simulink library "calcFluidDynamicLoads_hydroelasticVersion"  (R2022a)
settings: Solver=VariableStepAuto  StartTime=0.0  StopTime=10.0  RelTol=1e-3
values from neighbouring files (symbols this model uses):
  fluidDensity = 1000    [fluidDynamicSurface_ts.m]
undefined symbols (not defined in the file or in its folder): base_checkBending, base_checkTwisting, Copy_of_clAndCdCalculator_cl, E_matlabEnv, fluidMomentArms, fluidRefArea, G_matlabEnv, rho, Subsystem, vcl, vhcl, wingTips
libraries: dspstat3 x4, dsppolyfun x4, vrlib x3, dynamicPressure_ul x1, eeGeneralControl x1, alphaBetaLE_ul x1, localApparentWind_ul x1, rotateAboutVec x1, wingAnalysis_stateflow x1
settings Model: Creator=Ayaz  LastModifiedBy=Carson
settings SolverCC: AlgebraicLoopSolver=TrustRegion
settings DebuggingCC: UnconnectedInputMsg=warning  UnconnectedOutputMsg=warning  UnconnectedLineMsg=warning  SFMachineParentedDataDiag=warning

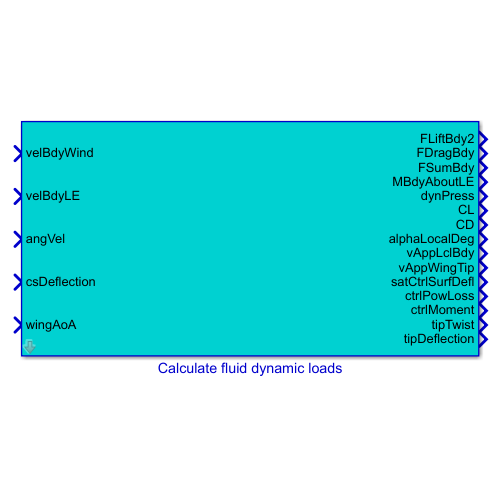
[thumbnail: Simulink's stored preview of the top-level diagram]
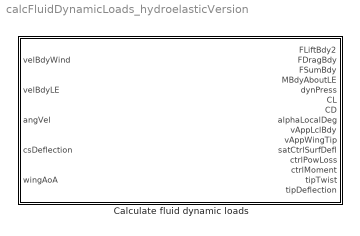
== system calcFluidDynamicLoads_hydroelasticVersion ==
  Calculate fluid dynamic loads : Subsystem  mask{aSurf=vcl.portWing, sRef=fluidRefArea, rArm_LE=fluidMomentArms(:,1), rTip_LE=wingTips(:,1), fluidDensity=fluidDensity}
      mask prompts: aSurf "Aerosurf object"; sRef "Reference area"; rArm_LE "Moment arm wrt wing LE"; rTip_LE "Surface tip wrt wing LE"; fluidDensity "Fluid density"

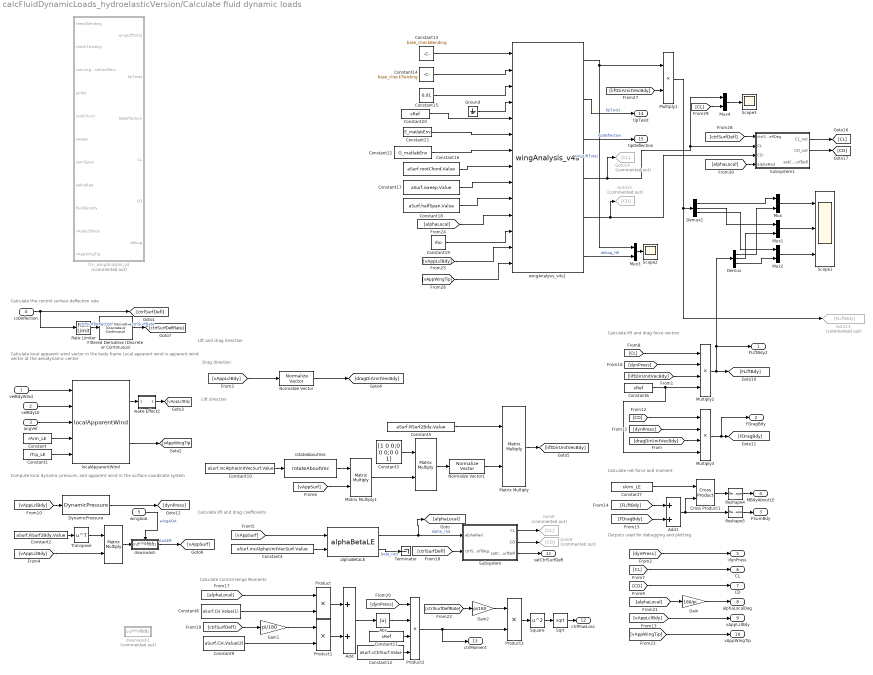
== system calcFluidDynamicLoads_hydroelasticVersion/Calculate fluid dynamic loads ==
  note: Calculate Control Hinge Moments
  note: Calculate the control surface deflection rate
  note: Lift and drag direction
  note: Lift direction
  note: Drag direction
  note: Compute local dynamic pressure,
      | and apparent wind in the surface coordinate system
  note: Calculate local apparent wind vector in the body frame
      | Local apparent wind is apparent wind vector at the aerodynamic center
  note: Calculate lift and drag coefficients
  note: Calculate net force and moment
  note: Outputs used for debugging and plotting.
  note: Calculate lift and drag force vectors
  velBdyWind : Inport
  velBdyLE : Inport  Port=2
  angVel : Inport  Port=3
  csDeflection : Inport  Port=4
  wingAoA : Inport  Port=5
  " " : Product  Multiplication=Matrix(*)
  "  " : Product  Multiplication=Matrix(*)
  Abs : Abs  SaturateOnIntegerOverflow=off
  Add : Sum
  Add1 : Sum
  Constant : Constant  Value=rArm_LE  VectorParams1D=off
  Constant1 : Constant  Value=rTip_LE  VectorParams1D=off
  Constant10 : Constant  Value=aSurf.incAlphaUnitVecSurf.Value  VectorParams1D=off
  Constant11 : Constant  Value=sRef
  Constant12 : Constant  Value=aSurf.cCtrlSurf.Value
  Constant13 : Constant  Value=base_checkBending  OutDataTypeStr=boolean
  Constant14 : Constant  Value=base_checkTwisting  OutDataTypeStr=boolean
  Constant15 : Constant  Value=0.01  OutDataTypeStr=double
  Constant16 : Constant  Value=aSurf.rootChord.Value
  Constant17 : Constant  Value=aSurf.sweep.Value
  Constant18 : Constant  Value=aSurf.halfSpan.Value
  Constant19 : Constant  Value=rho
  Constant2 : Constant  Value=aSurf.RSurf2Bdy.Value  VectorParams1D=off
  Constant20 : Constant  Value=sRef
  Constant21 : Constant  Value=E_matlabEnv
  Constant22 : Constant  Value=G_matlabEnv
  Constant3 : Constant  Value=[1 0 0;0 0 0;0 0 1]  VectorParams1D=off
  Constant4 : Constant  Value=aSurf.incAlphaUnitVecSurf.Value  VectorParams1D=off
  Constant5 : Constant  Value=aSurf.RSurf2Bdy.Value  VectorParams1D=off
  Constant6 : Constant  Value=sRef
  Constant7 : Constant  Value=rArm_LE  VectorParams1D=off
  Constant8 : Constant  Value=aSurf.CH.Value(1)
  Constant9 : Constant  Value=aSurf.CH.Value(2)
  Cross Product1 : vrlib/Utilities/Cross Product
  Demux : Demux  Outputs=3
  Demux1 : Demux  Outputs=3
  DynamicPressure : dynamicPressure_ul/DynamicPressure  rho=fluidDensity
  Filtered Derivative (Discrete or Continuous) : eeGeneralControl/Filtered Derivative (Discrete or Continuous)  K=1  T=.001  B=inf  A=-inf  minRatio=10  init_option=Inherited from block input  x0=0  Ts=-1
      settings: SourceProductBaseCode=PS
  Gain : Gain  Gain=180/pi
  Gain1 : Gain  Gain=pi/180
  Gain2 : Gain  Gain=pi/180
  Goto13 : Goto  Commented=on  GotoTag=FLiftBdy
  Goto14 : Goto  Commented=on  GotoTag=CL
  Goto15 : Goto  Commented=on  GotoTag=CD
  Goto8 : Goto  Commented=on  GotoTag=CL
  Goto9 : Goto  Commented=on  GotoTag=CD
  Ground : Ground
  Matrix Multiply : Product  Multiplication=Matrix(*)
  Matrix Multiply1 : Product  Multiplication=Matrix(*)
  Multiply1 : Product
  Multiply2 : Product  Inputs=4
  Multiply3 : Product  Inputs=4
  Mux{,1..4} (5 alike) : Mux  Inputs=2
  Normalize Vector : vrlib/Utilities/Normalize Vector  maxzero=0
  Normalize Vector1 : vrlib/Utilities/Normalize Vector  maxzero=0
  Product : Product
  Product1 : Product
  Product2 : Product  Inputs=4
  Product3 : Product
  Rate Limiter : RateLimiter  RisingSlewLimit=aSurf.maxCtrlDefSpeed.Value  FallingSlewLimit=-aSurf.maxCtrlDefSpeed.Value  SampleTimeMode=inherited
  Reshape4 : Reshape  OutputDimensionality=Column vector (2-D)
  Reshape5 : Reshape  OutputDimensionality=Column vector (2-D)
  Scope1 : Scope  NumInputPorts=3
  Scope2 : Scope
  Scope3 : Scope
  Sqrt : Sqrt
  Square : Math  Operator=square
  Subsystem : Subsystem  AncestorBlock=Copy_of_clAndCdCalculator_cl/Subsystem  mask{aSurf=aSurf}
      mask prompts: aSurf "aeroSurf object"
  Subsystem1 : Subsystem  mask{aSurf=aSurf}
      mask prompts: aSurf "aeroSurf object"
  Terminator : Terminator
  Transpose : Math  Operator=transpose  SignedPower=on
  alphaBetaLE : alphaBetaLE_ul/alphaBetaLE  SystemSampleTime=-1  VariantActivationTime=update diagram  Latency=0  AutoFrameSizeCalculation=off
  downwash : Subsystem
      settings: PortSchema="{\"entries\":[{\"content\":{\"sides\":[{\"content\":{\"connectorIds\":[\"In1\"]},\"type\":\"ConnectorPlacement.EquallySpacedRectSide\",\"uuid\":\"04ef6d2a-4770-4c63-9c45-9df535824cb6\"},{\"content\":{\"connectorIds\":[\"Out1\"],\"side\":\"RIGHT\"},\"type\":\"ConnectorPlacement.EquallySpacedRectSide\",\"uuid\":\"1e7f53a7-5f70-4bf0-8214-dce734c1b44e\"},{\"content\":{\"connectorIds\":[\"In2\"],\"side\":\"TOP\"},\"type\":\"ConnectorPlacement.EquallySpacedRectSide\",\"uuid\":\"18f507fa-715b-4755-b9b5-759b08e40168\"}]},\"type\":\"ConnectorPlacement.EquallySpacedConnector\",\"uuid\":\"684cff60-c972-427b-b388-36808b9016c1\"}],\"packageUris\":[\"http://schema.mathworks.com/mf0/Connector/19700101\"],\"version\":\"1.0\"}"
  downwash1 : Subsystem  Commented=on
      settings: PortSchema="{\"entries\":[{\"content\":{\"sides\":[{\"content\":{\"connectorIds\":[\"In1\"]},\"type\":\"ConnectorPlacement.EquallySpacedRectSide\",\"uuid\":\"04ef6d2a-4770-4c63-9c45-9df535824cb6\"},{\"content\":{\"connectorIds\":[\"Out1\"],\"side\":\"RIGHT\"},\"type\":\"ConnectorPlacement.EquallySpacedRectSide\",\"uuid\":\"1e7f53a7-5f70-4bf0-8214-dce734c1b44e\"},{\"content\":{\"connectorIds\":[\"In2\"],\"side\":\"TOP\"},\"type\":\"ConnectorPlacement.EquallySpacedRectSide\",\"uuid\":\"18f507fa-715b-4755-b9b5-759b08e40168\"}]},\"type\":\"ConnectorPlacement.EquallySpacedConnector\",\"uuid\":\"684cff60-c972-427b-b388-36808b9016c1\"}],\"packageUris\":[\"http://schema.mathworks.com/mf0/Connector/19700101\"],\"version\":\"1.0\"}"
  fcn_wingAnalysis_v4 : MATLAB Function  Commented=on  TreatAsAtomicUnit=on  SystemSampleTime=0.1
  localApparentWind : localApparentWind_ul/localApparentWind  SystemSampleTime=-1  VariantActivationTime=update diagram  Latency=0  AutoFrameSizeCalculation=off
  rotateAboutVec : rotateAboutVec/rotateAboutVec  ang=90
  wake Effect2 : Subsystem
  wingAnalysis_v4s1 : wingAnalysis_stateflow/wingAnalysis_v4s  SystemSampleTime=-1  VariantActivationTime=update diagram  Latency=0  AutoFrameSizeCalculation=off
      settings: PortSchema="{\"entries\":[{\"content\":{\"sides\":[{\"content\":{\"connectorIds\":[\"In1\",\"In2\",\"In3\",\"In11\",\"In12\",\"In13\",\"In14\",\"In4\",\"In5\",\"In6\",\"In7\",\"In8\",\"In9\",\"In10\"]},\"type\":\"ConnectorPlacement.EquallySpacedRectSide\",\"uuid\":\"6c729b90-d4cd-42cb-9ba5-b5252b1be0f3\"},{\"content\":{\"connectorIds\":[\"Out1\",\"Out2\",\"Out3\",\"Out4\",\"Out5\",\"Out6\"],\"side\":\"RIGHT\"},\"type\":\"ConnectorPlacement.EquallySpacedRectSide\",\"uuid\":\"eea762ff-71d7-4c66-90ee-932d903c73e3\"},{\"content\":{\"connectorIds\":[],\"side\":\"TOP\"},\"type\":\"ConnectorPlacement.EquallySpacedRectSide\",\"uuid\":\"df2db980-21fc-49eb-9688-a3d788e0d700\"}]},\"type\":\"ConnectorPlacement.EquallySpacedConnector\",\"uuid\":\"bf53f703-2290-4676-ac3c-dcfa73901a98\"}],\"packageUris\":[\"http://schema.mathworks.com/mf0/Connector/R2020b\"],\"version\":\"1.0\"}"
  FLiftBdy2 : Outport  VectorParamsAs1DForOutWhenUnconnected=off
  FDragBdy : Outport  Port=2  VectorParamsAs1DForOutWhenUnconnected=off
  FSumBdy : Outport  Port=3  VectorParamsAs1DForOutWhenUnconnected=off
  MBdyAboutLE : Outport  Port=4  PortDimensions=[3 1]  VectorParamsAs1DForOutWhenUnconnected=off
  dynPress : Outport  Port=5  VectorParamsAs1DForOutWhenUnconnected=off
  CL : Outport  Port=6  VectorParamsAs1DForOutWhenUnconnected=off
  CD : Outport  Port=7  VectorParamsAs1DForOutWhenUnconnected=off
  alphaLocalDeg : Outport  Port=8  VectorParamsAs1DForOutWhenUnconnected=off
  vAppLclBdy : Outport  Port=9  VectorParamsAs1DForOutWhenUnconnected=off
  vAppWingTip : Outport  Port=10  VectorParamsAs1DForOutWhenUnconnected=off
  satCtrlSurfDefl : Outport  Port=11
  ctrlPowLoss : Outport  Port=12
  ctrlMoment : Outport  Port=13
  tipTwist : Outport  Port=14
  tipDeflection : Outport  Port=15
  wires:
  Mux3/1 -> Scope2/1
  wingAnalysis_v4s1/6 -> Mux3/2  "debug_HE"
  wingAnalysis_v4s1/3 -> tipDeflection/1  "tipDeflection"
  wingAnalysis_v4s1/2 -> tipTwist/1  "tipTwist"
  Demux/3 -> Mux2/2
  Demux1/3 -> Mux2/1
  Demux/2 -> Mux1/2
  Demux1/2 -> Mux1/1
  Demux/1 -> Mux/2
  Demux1/1 -> Mux/1
  Mux2/1 -> Scope1/3
  Mux1/1 -> Scope1/2
  Mux/1 -> Scope1/1
  [liftDirUnitVecBdy] -> Multiply1/2
  wingAnalysis_v4s1/1 -> Multiply1/1, Mux3/1  "wingLiftTotal"
  [vAppWingTip] -> wingAnalysis_v4s1/10
  Constant15/1 -> wingAnalysis_v4s1/3
  Constant14/1 -> wingAnalysis_v4s1/2
  Constant13/1 -> wingAnalysis_v4s1/1
  velBdyLE/1 -> localApparentWind/2
  angVel/1 -> localApparentWind/3
  Constant/1 -> localApparentWind/4
  Constant1/1 -> localApparentWind/5
  Constant2/1 -> Transpose/1
  Transpose/1 -> "  "/1
  Constant3/1 -> " "/1
  rotateAboutVec/1 -> Matrix Multiply1/1
  Matrix Multiply/1 -> [liftDirUnitVecBdy]
  Normalize Vector1/1 -> Matrix Multiply/2
  Constant10/1 -> rotateAboutVec/1
  Matrix Multiply1/1 -> " "/2
  " "/1 -> Normalize Vector1/1
  Constant5/1 -> Matrix Multiply/1
  [vAppSurf] -> Matrix Multiply1/2
  Normalize Vector/1 -> [dragDirUnitVecBdy]
  [vAppLclBdy] -> Normalize Vector/1
  Constant4/1 -> alphaBetaLE/2
  Subsystem/2(CD) -> Goto9/1
  alphaBetaLE/2 -> Terminator/1  "beta_rad"
  [ctrlSurfDefl] -> Subsystem/2(ctrlSurfDeflDeg)
  Subsystem/1(CL) -> Goto8/1
  Constant6/1 -> Multiply2/4, Multiply3/4
  [vAppLclBdy] -> vAppLclBdy/1
  [dynPress] -> dynPress/1
  [FLiftBdy] -> Add1/1
  [vAppWingTip] -> vAppWingTip/1
  Multiply3/1 -> [FDragBdy], FDragBdy/1
  [dragDirUnitVecBdy] -> Multiply3/3
  [CD] -> CD/1
  [dynPress] -> Multiply2/2
  [alphaLocal] -> Gain/1
  [dynPress] -> Multiply3/2
  [CL] -> CL/1
  [CL] -> Multiply2/1
  [liftDirUnitVecBdy] -> Multiply2/3
  Multiply2/1 -> Demux/1, FLiftBdy2/1, [FLiftBdy]
  [CD] -> Multiply3/1
  [FDragBdy] -> Add1/2
  Reshape5/1 -> FSumBdy/1
  Cross Product1/1 -> Reshape4/1
  Add1/1 -> Cross Product1/2, Reshape5/1
  Constant7/1 -> Cross Product1/1
  Gain/1 -> alphaLocalDeg/1
  Reshape4/1 -> MBdyAboutLE/1
  Filtered Derivative (Discrete or Continuous)/1 -> [ctrlSurfDeflRate]  "ctrlSurfRate"
  [alphaLocal] -> Product/1
  Constant8/1 -> Product/2
  [ctrlSurfDefl] -> Gain1/1
  Constant9/1 -> Product1/2
  Product1/1 -> Add/2
  Product/1 -> Add/1
  Add/1 -> Abs/1
  [dynPress] -> Product2/1
  Constant11/1 -> Product2/3
  Constant12/1 -> Product2/4
  Product2/1 -> ctrlMoment/1, Product3/2
  [ctrlSurfDeflRate] -> Gain2/1
  Abs/1 -> Product2/2
  Gain1/1 -> Product1/1
  Gain2/1 -> Product3/1
  csDeflection/1 -> Rate Limiter/1, [ctrlSurfDefl]
  Rate Limiter/1 -> Filtered Derivative (Discrete or Continuous)/1  "ctrlSurfDeflection"
  Product3/1 -> Square/1
  Square/1 -> Sqrt/1
  Sqrt/1 -> ctrlPowLoss/1
  [vAppSurf] -> alphaBetaLE/1
  localApparentWind/2 -> [vAppWingTip]
  [vAppLclBdy] -> DynamicPressure/1
  [vAppLclBdy] -> "  "/2
  DynamicPressure/1 -> [dynPress]
  velBdyWind/1 -> localApparentWind/1
  localApparentWind/1 -> wake Effect2/1(velWindBdy)
  wake Effect2/1(Out1) -> [vAppLclBdy]
  downwash/1(Out1) -> [vAppSurf]  "AoAEff"
  "  "/1 -> downwash/1(In1)
  alphaBetaLE/1 -> Subsystem/1(alphaRad), [alphaLocal]  "alpha_rad"
  wingAoA/1 -> downwash/2(wingAoA)  "wingAOA"
  Multiply1/1 -> Goto13/1, Demux1/1
  wingAnalysis_v4s1/4 -> Goto14/1, Mux4/1, Subsystem1/2(CL)
  wingAnalysis_v4s1/5 -> Goto15/1, Subsystem1/3(CD)
  Constant16/1 -> wingAnalysis_v4s1/4
  Constant17/1 -> wingAnalysis_v4s1/5
  Constant18/1 -> wingAnalysis_v4s1/6
  [alphaLocal] -> wingAnalysis_v4s1/7
  Constant19/1 -> wingAnalysis_v4s1/8
  [vAppLclBdy] -> wingAnalysis_v4s1/9
  Ground/1 -> wingAnalysis_v4s1/11
  [ctrlSurfDefl] -> Subsystem1/1(ctrlSurfDeflDeg)
  Subsystem1/1(CL_out) -> [CL]
  Subsystem1/2(CD_out) -> [CD]
  Subsystem/3(satCtrlSurfDefl) -> satCtrlSurfDefl/1
  Mux4/1 -> Scope3/1
  [CL] -> Mux4/2
  [alphaLocal] -> Subsystem1/4(alphaRad)
  Constant20/1 -> wingAnalysis_v4s1/12
  Constant21/1 -> wingAnalysis_v4s1/13
  Constant22/1 -> wingAnalysis_v4s1/14

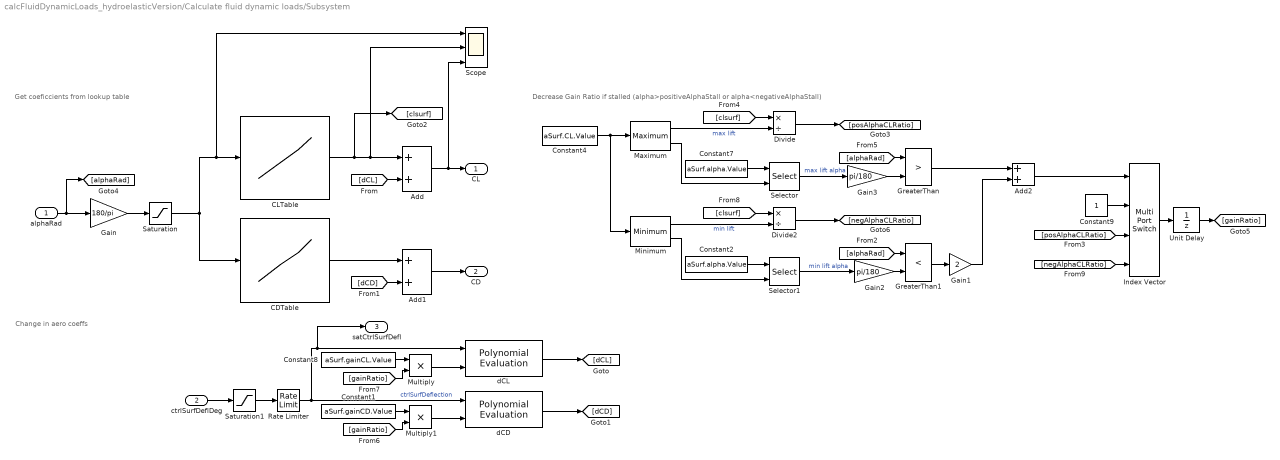
== system calcFluidDynamicLoads_hydroelasticVersion/Calculate fluid dynamic loads/Subsystem ==
  note: Get coeficcients from lookup table
  note: Change in aero coeffs
  note: Decrease Gain Ratio if stalled (alpha>positiveAlphaStall or alpha<negativeAlphaStall)
  alphaRad : Inport
  ctrlSurfDeflDeg : Inport  Port=2
  Add : Sum
  Add1 : Sum
  Add2 : Sum
  CDTable : Lookup_n-D  NumberOfTableDimensions=1  LookupTableObject=CLTable  BreakpointsForDimension1=aSurf.alpha.Value  Table=aSurf.CD.Value  ExtrapMethod=Clip  UseLastTableValue=on  InternalRulePriority=Speed  RndMeth=Simplest
  CLTable : Lookup_n-D  NumberOfTableDimensions=1  LookupTableObject=CLTable  BreakpointsForDimension1=aSurf.alpha.Value  Table=aSurf.CL.Value  ExtrapMethod=Clip  UseLastTableValue=on  InternalRulePriority=Speed  RndMeth=Simplest
  Constant1 : Constant  Value=aSurf.gainCD.Value
  Constant2 : Constant  Value=aSurf.alpha.Value
  Constant4 : Constant  Value=aSurf.CL.Value
  Constant7 : Constant  Value=aSurf.alpha.Value
  Constant8 : Constant  Value=aSurf.gainCL.Value
  Constant9 : Constant
  Divide : Product  Inputs=*/
  Divide2 : Product  Inputs=*/
  Gain : Gain  Gain=180/pi
  Gain1 : Gain  Gain=2
  Gain2 : Gain  Gain=pi/180
  Gain3 : Gain  Gain=pi/180
  GreaterThan : RelationalOperator  Operator=>  OutDataTypeStr=boolean  RndMeth=Simplest  InputSameDT=off
  GreaterThan1 : RelationalOperator  Operator=<  OutDataTypeStr=boolean  RndMeth=Simplest  InputSameDT=off
  Index Vector : MultiPortSwitch  DataPortOrder=Zero-based contiguous  zeroidx=on  SaturateOnIntegerOverflow=off  InputSameDT=off
  Maximum : dspstat3/Maximum  operation=maximum  fcn=Value and Index  indexBase=One  operateOver=Each column  Dimension=1  InputProcessing=Columns as channels (frame based)  reset=None  roiEnable=off  roiType=Rectangles  roiPortion=Entire ROI  roiOutput=Individual statistics for each ROI  roiFlag=off  roundingMode=Floor  overflowMode=off  accumDataTypeStr=Inherit: Same as product output  accumLastDataTypeStr=Inherit: Same as product output
  Minimum : dspstat3/Minimum  operation=minimum  fcn=Value and Index  indexBase=One  operateOver=Each column  Dimension=1  InputProcessing=Columns as channels (frame based)  reset=None  roiEnable=off  roiType=Rectangles  roiPortion=Entire ROI  roiOutput=Individual statistics for each ROI  roiFlag=off  roundingMode=Floor  overflowMode=off
      settings: SourceProductBaseCode=DS
  Multiply : Product
  Multiply1 : Product
  Rate Limiter : RateLimiter  RisingSlewLimit=aSurf.maxCtrlDefSpeed.Value  FallingSlewLimit=-aSurf.maxCtrlDefSpeed.Value  SampleTimeMode=inherited
  Saturation : Saturate  UpperLimit=90  LowerLimit=-90
  Saturation1 : Saturate  UpperLimit=aSurf.maxCtrlDef.Value  LowerLimit=aSurf.minCtrlDef.Value
  Scope : Scope  NumInputPorts=3
  Selector : Selector  InputPortWidth=length(vhcl.portWing.alpha.Value)  IndexOptions=Index vector (port)  Indices=[1 3]  OutputSizes=1
  Selector1 : Selector  InputPortWidth=length(vhcl.portWing.alpha.Value)  IndexOptions=Index vector (port)  Indices=[1 3]  OutputSizes=1
  Unit Delay : UnitDelay  InitialCondition=1  SampleTime=-1  HasFrameUpgradeWarning=on
  dCD : dsppolyfun/Polynomial Evaluation  useConstCoeffs=off  constCoeffs=[0]
      settings: SourceProductBaseCode=DS
  dCL : dsppolyfun/Polynomial Evaluation  useConstCoeffs=off  constCoeffs=[0]
      settings: SourceProductBaseCode=DS
  CL : Outport  VectorParamsAs1DForOutWhenUnconnected=off
  CD : Outport  Port=2  VectorParamsAs1DForOutWhenUnconnected=off
  satCtrlSurfDefl : Outport  Port=3
  wires:
  Add2/1 -> Index Vector/1
  Constant1/1 -> Multiply1/1
  Gain2/1 -> GreaterThan1/2
  Maximum/2 -> Selector/2
  Multiply/1 -> dCL/2
  Constant9/1 -> Index Vector/2
  [gainRatio] -> Multiply/2
  [posAlphaCLRatio] -> Index Vector/3
  [dCL] -> Add/2
  [alphaRad] -> GreaterThan1/1
  [clsurf] -> Divide/1
  Maximum/1 -> Divide/2  "max lift"
  Selector1/1 -> Gain2/1  "min lift alpha"
  Divide2/1 -> [negAlphaCLRatio]
  Divide/1 -> [posAlphaCLRatio]
  Selector/1 -> Gain3/1  "max lift alpha"
  dCL/1 -> [dCL]
  [clsurf] -> Divide2/1
  Constant4/1 -> Minimum/1, Maximum/1
  dCD/1 -> [dCD]
  Minimum/2 -> Selector1/2
  GreaterThan1/1 -> Gain1/1
  CDTable/1 -> Add1/1
  Rate Limiter/1 -> dCD/1, satCtrlSurfDefl/1, dCL/1  "ctrlSurfDeflection"
  Saturation/1 -> CDTable/1, CLTable/1, Scope/1
  Constant2/1 -> Selector1/1
  Minimum/1 -> Divide2/2  "min lift"
  alphaRad/1 -> Gain/1, [alphaRad]
  Add/1 -> CL/1, Scope/3
  Constant8/1 -> Multiply/1
  [negAlphaCLRatio] -> Index Vector/4
  Gain/1 -> Saturation/1
  Gain3/1 -> GreaterThan/2
  ctrlSurfDeflDeg/1 -> Saturation1/1
  GreaterThan/1 -> Add2/1
  [alphaRad] -> GreaterThan/1
  Add1/1 -> CD/1
  Gain1/1 -> Add2/2
  CLTable/1 -> Add/1, Scope/2, [clsurf]
  Constant7/1 -> Selector/1
  Index Vector/1 -> Unit Delay/1
  [gainRatio] -> Multiply1/2
  Saturation1/1 -> Rate Limiter/1
  [dCD] -> Add1/2
  Multiply1/1 -> dCD/2
  Unit Delay/1 -> [gainRatio]

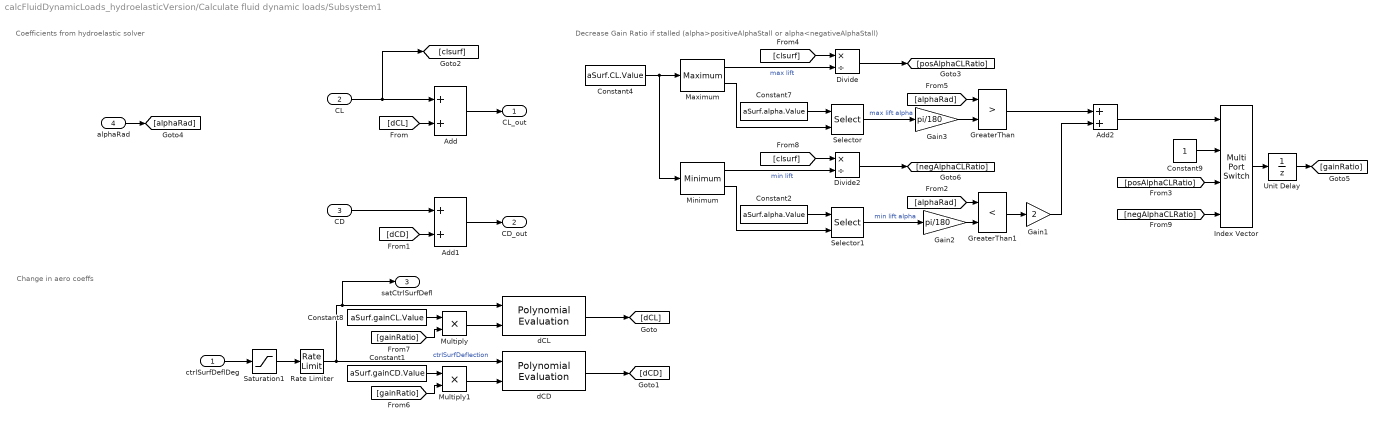
== system calcFluidDynamicLoads_hydroelasticVersion/Calculate fluid dynamic loads/Subsystem1 ==
  note: Decrease Gain Ratio if stalled (alpha>positiveAlphaStall or alpha<negativeAlphaStall)
  note: Change in aero coeffs
  note: Coefficients from hydroelastic solver
  ctrlSurfDeflDeg : Inport
  CL : Inport  Port=2
  CD : Inport  Port=3
  alphaRad : Inport  Port=4
  Add : Sum
  Add1 : Sum
  Add2 : Sum
  Constant1 : Constant  Value=aSurf.gainCD.Value
  Constant2 : Constant  Value=aSurf.alpha.Value
  Constant4 : Constant  Value=aSurf.CL.Value
  Constant7 : Constant  Value=aSurf.alpha.Value
  Constant8 : Constant  Value=aSurf.gainCL.Value
  Constant9 : Constant
  Divide : Product  Inputs=*/
  Divide2 : Product  Inputs=*/
  Gain1 : Gain  Gain=2
  Gain2 : Gain  Gain=pi/180
  Gain3 : Gain  Gain=pi/180
  GreaterThan : RelationalOperator  Operator=>  OutDataTypeStr=boolean  RndMeth=Simplest  InputSameDT=off
  GreaterThan1 : RelationalOperator  Operator=<  OutDataTypeStr=boolean  RndMeth=Simplest  InputSameDT=off
  Index Vector : MultiPortSwitch  DataPortOrder=Zero-based contiguous  zeroidx=on  SaturateOnIntegerOverflow=off  InputSameDT=off
  Maximum : dspstat3/Maximum  operation=maximum  fcn=Value and Index  indexBase=One  operateOver=Each column  Dimension=1  InputProcessing=Columns as channels (frame based)  reset=None  roiEnable=off  roiType=Rectangles  roiPortion=Entire ROI  roiOutput=Individual statistics for each ROI  roiFlag=off  roundingMode=Floor  overflowMode=off  accumDataTypeStr=Inherit: Same as product output  accumLastDataTypeStr=Inherit: Same as product output
  Minimum : dspstat3/Minimum  operation=minimum  fcn=Value and Index  indexBase=One  operateOver=Each column  Dimension=1  InputProcessing=Columns as channels (frame based)  reset=None  roiEnable=off  roiType=Rectangles  roiPortion=Entire ROI  roiOutput=Individual statistics for each ROI  roiFlag=off  roundingMode=Floor  overflowMode=off
      settings: SourceProductBaseCode=DS
  Multiply : Product
  Multiply1 : Product
  Rate Limiter : RateLimiter  RisingSlewLimit=aSurf.maxCtrlDefSpeed.Value  FallingSlewLimit=-aSurf.maxCtrlDefSpeed.Value  SampleTimeMode=inherited
  Saturation1 : Saturate  UpperLimit=aSurf.maxCtrlDef.Value  LowerLimit=aSurf.minCtrlDef.Value
  Selector : Selector  InputPortWidth=length(vhcl.portWing.alpha.Value)  IndexOptions=Index vector (port)  Indices=[1 3]  OutputSizes=1
  Selector1 : Selector  InputPortWidth=length(vhcl.portWing.alpha.Value)  IndexOptions=Index vector (port)  Indices=[1 3]  OutputSizes=1
  Unit Delay : UnitDelay  InitialCondition=1  SampleTime=-1  HasFrameUpgradeWarning=on
  dCD : dsppolyfun/Polynomial Evaluation  useConstCoeffs=off  constCoeffs=[0]
      settings: SourceProductBaseCode=DS
  dCL : dsppolyfun/Polynomial Evaluation  useConstCoeffs=off  constCoeffs=[0]
      settings: SourceProductBaseCode=DS
  CL_out : Outport  VectorParamsAs1DForOutWhenUnconnected=off
  CD_out : Outport  Port=2  VectorParamsAs1DForOutWhenUnconnected=off
  satCtrlSurfDefl : Outport  Port=3
  wires:
  Unit Delay/1 -> [gainRatio]
  Multiply1/1 -> dCD/2
  [dCD] -> Add1/2
  Saturation1/1 -> Rate Limiter/1
  [gainRatio] -> Multiply1/2
  Index Vector/1 -> Unit Delay/1
  Constant7/1 -> Selector/1
  CL/1 -> [clsurf], Add/1
  Gain1/1 -> Add2/2
  Add1/1 -> CD_out/1
  [alphaRad] -> GreaterThan/1
  GreaterThan/1 -> Add2/1
  ctrlSurfDeflDeg/1 -> Saturation1/1
  Gain3/1 -> GreaterThan/2
  [negAlphaCLRatio] -> Index Vector/4
  Constant8/1 -> Multiply/1
  Add/1 -> CL_out/1
  Minimum/1 -> Divide2/2  "min lift"
  Constant2/1 -> Selector1/1
  Rate Limiter/1 -> dCL/1, satCtrlSurfDefl/1, dCD/1  "ctrlSurfDeflection"
  CD/1 -> Add1/1
  GreaterThan1/1 -> Gain1/1
  Minimum/2 -> Selector1/2
  dCD/1 -> [dCD]
  Constant4/1 -> Maximum/1, Minimum/1
  [clsurf] -> Divide2/1
  dCL/1 -> [dCL]
  Selector/1 -> Gain3/1  "max lift alpha"
  Divide/1 -> [posAlphaCLRatio]
  Divide2/1 -> [negAlphaCLRatio]
  Selector1/1 -> Gain2/1  "min lift alpha"
  Maximum/1 -> Divide/2  "max lift"
  [clsurf] -> Divide/1
  [alphaRad] -> GreaterThan1/1
  [dCL] -> Add/2
  [posAlphaCLRatio] -> Index Vector/3
  [gainRatio] -> Multiply/2
  Constant9/1 -> Index Vector/2
  Multiply/1 -> dCL/2
  Maximum/2 -> Selector/2
  Gain2/1 -> GreaterThan1/2
  Constant1/1 -> Multiply1/1
  Add2/1 -> Index Vector/1
  alphaRad/1 -> [alphaRad]

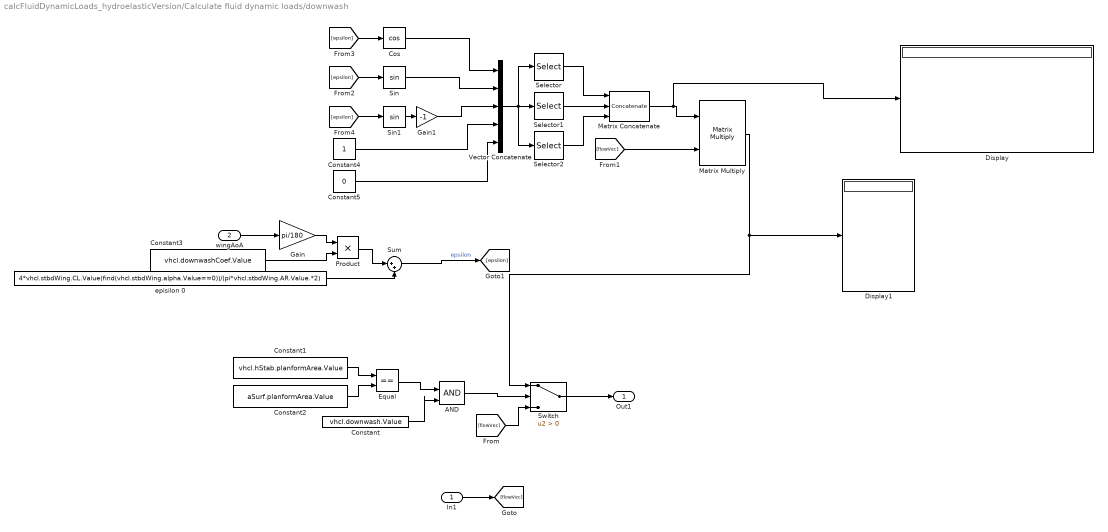
== system calcFluidDynamicLoads_hydroelasticVersion/Calculate fluid dynamic loads/downwash ==
  In1 : Inport
  wingAoA : Inport  Port=2
  AND : Logic  IconShape=distinctive  AllPortsSameDT=off  OutDataTypeStr=boolean
  Constant : Constant  Value=vhcl.downwash.Value
  Constant1 : Constant  Value=vhcl.hStab.planformArea.Value
  Constant2 : Constant  Value=aSurf.planformArea.Value
  Constant3 : Constant  Value=vhcl.downwashCoef.Value
  Constant4 : Constant
  Constant5 : Constant  Value=0
  Cos : Trigonometry  Operator=cos
  Display : Display
  Display1 : Display
  Equal : RelationalOperator  Operator===  OutDataTypeStr=boolean  RndMeth=Simplest  InputSameDT=off
  Gain : Gain  Gain=pi/180
  Gain1 : Gain  Gain=-1
  Matrix Concatenate : Concatenate  NumInputs=3  Mode=Multidimensional array  ConcatenateDimension=2
  Matrix Multiply : Product  Multiplication=Matrix(*)
  Product : Product
  Selector : Selector  InputPortWidth=5  IndexOptions=Index vector (dialog)  Indices=[1 5 3]  OutputSizes=1
  Selector1 : Selector  InputPortWidth=5  IndexOptions=Index vector (dialog)  Indices=[5 4 5]  OutputSizes=1
  Selector2 : Selector  InputPortWidth=5  IndexOptions=Index vector (dialog)  Indices=[2 5 1]  OutputSizes=1
  Sin : Trigonometry
  Sin1 : Trigonometry
  Sum : Sum  Inputs=|++
  Switch : Switch  Criteria=u2 > Threshold  SaturateOnIntegerOverflow=off  InputSameDT=off
  Vector Concatenate : Concatenate  NumInputs=5
  episilon 0 : Constant  Value=4*vhcl.stbdWing.CL.Value(find(vhcl.stbdWing.alpha.Value==0))/(pi*vhcl.stbdWing.AR.Value.*2)
  Out1 : Outport
  wires:
  Switch/1 -> Out1/1
  Constant1/1 -> Equal/1
  Constant2/1 -> Equal/2
  Equal/1 -> AND/1
  Constant/1 -> AND/2
  AND/1 -> Switch/2
  In1/1 -> [flowVec]
  [flowVec] -> Switch/3
  Constant3/1 -> Product/2
  Product/1 -> Sum/1
  [flowVec] -> Matrix Multiply/2
  episilon 0/1 -> Sum/2
  Matrix Multiply/1 -> Switch/1, Display1/1
  Gain/1 -> Product/1
  wingAoA/1 -> Gain/1
  [epsilon] -> Sin/1
  [epsilon] -> Cos/1
  [epsilon] -> Sin1/1
  Sin1/1 -> Gain1/1
  Constant4/1 -> Vector Concatenate/4
  Gain1/1 -> Vector Concatenate/3
  Sin/1 -> Vector Concatenate/2
  Cos/1 -> Vector Concatenate/1
  Vector Concatenate/1 -> Selector2/1, Selector1/1, Selector/1
  Constant5/1 -> Vector Concatenate/5
  Selector2/1 -> Matrix Concatenate/3
  Selector1/1 -> Matrix Concatenate/2
  Selector/1 -> Matrix Concatenate/1
  Matrix Concatenate/1 -> Display/1, Matrix Multiply/1
  Sum/1 -> [epsilon]  "epsilon"

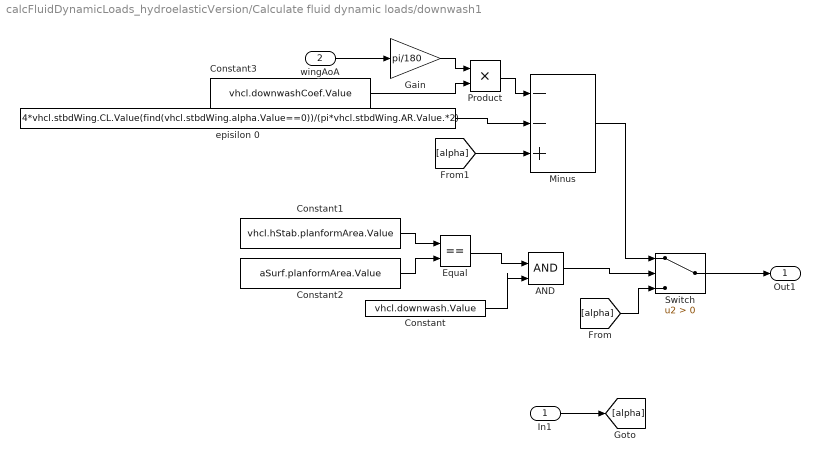
== system calcFluidDynamicLoads_hydroelasticVersion/Calculate fluid dynamic loads/downwash1 ==
  In1 : Inport
  wingAoA : Inport  Port=2
  AND : Logic  IconShape=distinctive  AllPortsSameDT=off  OutDataTypeStr=boolean
  Constant : Constant  Value=vhcl.downwash.Value
  Constant1 : Constant  Value=vhcl.hStab.planformArea.Value
  Constant2 : Constant  Value=aSurf.planformArea.Value
  Constant3 : Constant  Value=vhcl.downwashCoef.Value
  Equal : RelationalOperator  Operator===  OutDataTypeStr=boolean  RndMeth=Simplest  InputSameDT=off
  Gain : Gain  Gain=pi/180
  Minus : Sum  Inputs=--+
  Product : Product
  Switch : Switch  Criteria=u2 > Threshold  SaturateOnIntegerOverflow=off  InputSameDT=off
  episilon 0 : Constant  Value=4*vhcl.stbdWing.CL.Value(find(vhcl.stbdWing.alpha.Value==0))/(pi*vhcl.stbdWing.AR.Value.*2)
  Out1 : Outport
  wires:
  Switch/1 -> Out1/1
  Constant1/1 -> Equal/1
  Constant2/1 -> Equal/2
  Equal/1 -> AND/1
  Constant/1 -> AND/2
  AND/1 -> Switch/2
  In1/1 -> [alpha]
  [alpha] -> Switch/3
  Constant3/1 -> Product/2
  Product/1 -> Minus/1
  [alpha] -> Minus/3
  episilon 0/1 -> Minus/2
  Minus/1 -> Switch/1
  Gain/1 -> Product/1
  wingAoA/1 -> Gain/1

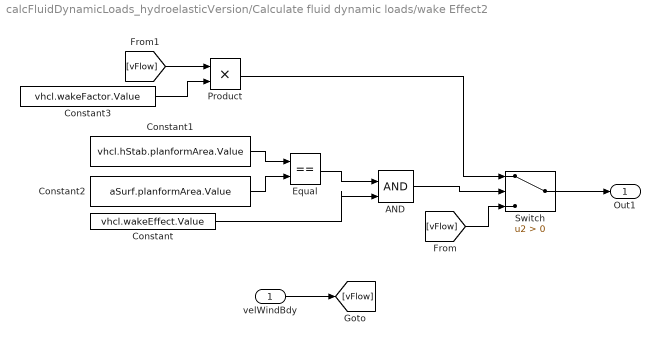
== system calcFluidDynamicLoads_hydroelasticVersion/Calculate fluid dynamic loads/wake Effect2 ==
  velWindBdy : Inport
  AND : Logic  IconShape=distinctive  AllPortsSameDT=off  OutDataTypeStr=boolean
  Constant : Constant  Value=vhcl.wakeEffect.Value
  Constant1 : Constant  Value=vhcl.hStab.planformArea.Value
  Constant2 : Constant  Value=aSurf.planformArea.Value
  Constant3 : Constant  Value=vhcl.wakeFactor.Value
  Equal : RelationalOperator  Operator===  OutDataTypeStr=boolean  RndMeth=Simplest  InputSameDT=off
  Product : Product
  Switch : Switch  Criteria=u2 > Threshold  SaturateOnIntegerOverflow=off  InputSameDT=off
  Out1 : Outport
  wires:
  Constant/1 -> AND/2
  [vFlow] -> Switch/3
  [vFlow] -> Product/1
  Equal/1 -> AND/1
  velWindBdy/1 -> [vFlow]
  Constant2/1 -> Equal/2
  Constant1/1 -> Equal/1
  AND/1 -> Switch/2
  Constant3/1 -> Product/2
  Product/1 -> Switch/1
  Switch/1 -> Out1/1

== matlab function calcFluidDynamicLoads_hydroelasticVersion/Calculate fluid dynamic loads/fcn_wingAnalysis_v4 ==
  data: checkBending input boolean size=1; wingLiftTotal output size=1; checkTwisting input boolean size=1; convergenceGoalPerc input size=1; airfoil input size=1; rootChord input size=1; sweep input size=1; semiSpan input size=1; alphaRad input size=1; fluidDensity input size=1; vAppLclBody input size=[3 1]; vAppWingTip input size=[3 1]; tipTwist output size=1; tipDeflection output size=1; CL output size=1; CD output size=1; debug output size=1
function [wingLiftTotal, tipTwist, tipDeflection, CL, CD, debug] = fcn_wingAnalysis_v4(checkBending, checkTwisting, convergenceGoalPerc, airfoil, rootChord, sweep, ...
    semiSpan, alphaRad, fluidDensity, vAppLclBody, vAppWingTip)

persistent F_cl
persistent F_cd
persistent F_cm
persistent F_alfaCl
persistent wingMatLast
coder.extrinsic('scatteredInterpolant') % therefore this function will not work if code is compiled
coder.extrinsic('griddedInterpolant')

if isempty(F_cl)
    combData = load('combinedMat_20220915.mat');
    combData = combData.combData;
    F_cl = scatteredInterpolant(combData(:,1), combData(:,2), combData(:,3)); % Cl = F_cl(Re, alfa)
    F_cd = scatteredInterpolant(combData(:,1), combData(:,2), combData(:,4)); % Cd = F_cl(Re, alfa)
    F_cm = scatteredInterpolant(combData(:,1), combData(:,2), combData(:,6)); % Cm = F_cl(Re, alfa)
    F_alfaCl = scatteredInterpolant(combData(:,1), combData(:,3), combData(:,2)); % alfa = F_alfaCl(Re, Cl)
end

drawPlots = 0;
animateWing = 0;
writeDiagnostics = 0;
convergence_goal_perc = convergenceGoalPerc; % convergence criteria, percent difference between each element bending and twisting

%airfoil = 'NACA_2412';
%rootChord = 1; % m
%sweep = 2.3; % deg
wingLength = semiSpan; % m (half span)
tipChord = rootChord - wingLength*tand(sweep); % m
area = tipChord*wingLength + 0.5*(rootChord-tipChord)*wingLength;
AR = 2*wingLength^2 / area;
AoA = alphaRad*180/pi; % deg
%AoA = 2;
%re = 50000;
nu_water = 1.5217e-6; % m2/s, kinematic visc. water
rho = fluidDensity; % kg/m3 (water)
% wing starting twist would be cool, not needed for us

% beam approximation TODO
beamWidth = 0.037; % m
beamHeight = 0.1; % m
I = (1/12*beamWidth*beamHeight^3); % this needs to be updated at each node as that node twists
%E = 69e9; % modulus of elasticity, Al 6061
E = 20e9;
G = 26e9; % shear modulus, Al 6061

% setup wing matrix
numEl = 30; % node 0 is fixed point => numEl nodes that need evaluated
elLength = wingLength/numEl;
wingMat = zeros(numEl, 12); % [x z alpha chord flowVel lift moment drag alfaZeroLift lift_x lift_z twist] (lift_x = sideslip force)
%wingMat(:,1) = elLength:elLength:wingLength;
wingMat(:,1) = (linspace(elLength, wingLength, numEl))';
wingMat(:,3) = AoA; % AoA, degrees
wingMat(:,4) = (linspace(rootChord, tipChord, numEl))';
%wingMat(:,5) = wing_vel; % m/s, not in a turn
%wingMat(:,3) = linspace(0, 1, numEl); % for testing
%yawRate = yawRateIn; % rad/s
%wingMat(:,5) = wingMat(:,5) + yawRate.*wingMat(:,1); % add yaw rate
wingMat(:,5) = (linspace(vAppLclBody(1), vAppWingTip(1), numEl))';

c_m = nan(1);
c_d = nan(1);
alfaZL = nan(1);
wingLiftTotal = 0;
CL_LLT = nan(1);

done = 0;
for iteration = 1:15
    if ~done
        alpha_last = nan(1);
        %wbar = waitbar(0, 'Finding lift and moment at nodes');
        for q = 1:numEl
            alpha = wingMat(q,3);
            if q == 1 || alpha ~= alpha_last % need to check coeffs
                re = wingMat(q, 5) * wingMat(q,4) / nu_water;
                %re = 150000;
                %[c_l, c_d, c_m] = func_findAirfoilCoeff(airfoil, re, alpha);
                %c_l = F_cl(re, alpha);
                c_m = F_cm(re, alpha);
                c_d = F_cd(re, alpha);
                alfaZL = F_alfaCl(re, 0); % looks up airfoil alpha zero lift

                % 2D -> 3D coefficient corrections
                %c_L = c_l;% / (1+2/AR); only good for AR > 5
                %c_L = c_L + dCL; % from control surface
        
            else % alpha == alpha_last, no need to re-calc coeffs
            end
        
            Q = 0.5*rho*wingMat(q,5)^2; % freestream dynamic press
            %Q = dynPress;
            S = wingMat(q,4)*elLength; % element reference area 
            %wingMat(q,6) = c_L*Q*S; % lift at node 
            wingMat(q,7) = c_m*Q*S*wingMat(q,4); % moment at node
            wingMat(q,8) = c_d*Q*S*wingMat(q,4); % drag at node
            wingMat(q,9) = alfaZL;
            
            %waitbar(q/numEl, wbar);
            alpha_last = alpha;
        end
        % function func_LLT expects full wing
        wingVel = zeros(numEl*2, 1); % need to solve for fluid velocity of other side of wing
        wingVel(1:numEl) = (linspace(vAppLclBody(1) - (vAppWingTip(1) - vAppLclBody(1)), vAppLclBody(1), numEl))';
        wingVel(numEl+1:end) = wingMat(:,5);
        [loadMat, CL_LLT] = func_LLT([flipud(wingMat(:,3)); wingMat(:,3)], [flipud(-wingMat(:,1)); wingMat(:,1)], [flipud(wingMat(:,9)); wingMat(:,9)], ...
            [flipud(wingMat(:,4)); wingMat(:,4)], wingLength*2, [flipud(wingMat(:,12)); wingMat(:,12)], wingVel, rho, AR, 10);
        %close(wbar);
        wingMat(:,6) = loadMat(numEl+1:end, 2);

        %tempMat(end+1,:) = [CL_LLT*dynPress*area, sum(wingMat(:,6))*2];
        
        
        if checkBending
            bendMat = bendingFunc(wingMat(:,6), E, I, wingLength);
            wingMat(:,2) = bendMat(:,2);
        end
        
        
        if checkTwisting
            twistMat = twistingFunc(wingMat(:,7), beamWidth, beamHeight, G, wingLength, AoA*pi/180);
            wingMat(:,12) = twistMat(:,2) * 180/pi; % convert to deg
        end

        matMod = [0 0; wingMat(:,1:2)];
        wingMat(:,10) = wingMat(:,6).* sin(atan((matMod(2:end, 2) - matMod(1:end-1, 2))./(matMod(2:end, 1) - matMod(1:end-1, 1))));
        wingMat(:,11) = wingMat(:,6).* cos(atan((matMod(2:end, 2) - matMod(1:end-1, 2))./(matMod(2:end, 1) - matMod(1:end-1, 1))));
        
        if writeDiagnostics
            %fprintf('Iteration %.0f Max deflection = %.4f Max twist = %.4f\n', iteration, wingMat(end,2), wingMat(end,3));
        end
        
        if drawPlots    
            figure(20)
            hold on
            plot(wingMat(:,1), wingMat(:,2))
            axis equal
            figure(21)
            hold on
            plot(wingMat(:,1), wingMat(:,3))
        end
    
        if isempty(wingMatLast)
            wingMatLast = wingMat;
        else
            perDiff_defl = [abs(wingMat(:,2)-wingMatLast(:,2))]' ./ mean([wingMat(:,2), wingMatLast(:,2)]');
            if isnan(perDiff_defl)
                perDiff_defl = zeros(1,numEl);
            end
            perDiff_twst = [abs(wingMat(:,3)-wingMatLast(:,3))]' ./ mean([wingMat(:,3), wingMatLast(:,3)]');
            if isnan(perDiff_twst)
                perDiff_twst = zeros(1,numEl);
            end
    
            if mean(perDiff_defl) < convergence_goal_perc && mean(perDiff_twst) < convergence_goal_perc
                done = 1;
                if writeDiagnostics
                    fprintf('Converged in %.0f iterations\n', iteration);
                end
            end
            wingMatLast = wingMat;
            
        end
    end
end
wingLiftTotal = sum(wingMat(:,11));
tipTwist = wingMat(end,12);
tipDeflection = wingMat(end,2);
CL = CL_LLT/2; % report half wing CL
dragTotal = sum(wingMat(:,8));
Q_root = 0.5*rho*vAppLclBody(1)^2;
CD = dragTotal/Q_root/area;

debug = sum(wingMat(:,6));

if animateWing
    figure(20)
    xlim([0 5])
    plot(wingMat(:,1), wingMat(:,2), 'bo-')
    axis equal
    drawnow
end
end
